simulink model "ExportExample"  (Simulink 7.6)
settings: Solver=FixedStepDiscrete  SolverMode=SingleTasking  StartTime=0.0  StopTime=100.0  RelTol=1e-3
InitFcn:
  | %% DSPBuilder Start
  | alt_dspbuilder_update_model(bdroot)
  | %% DSPBuilder End
libraries: allblocks_alteradspbuilder2 x8
settings Model: Creator=gnixon  LastModifiedBy=akarapet
settings OptimizationCC: InlineInvariantSignals=on  InitFltsAndDblsToZero=on
settings DebuggingCC: SaveWithParameterizedLinksMsg=none  SignalResolutionControl=TryResolveAllWithWarning  SolverPrmCheckMsg=none  MultiTaskDSMMsg=warning  MultiTaskCondExecSysMsg=none  StrictBusMsg=Warning
settings HardwareCC: TargetUnknown=on
settings RTWCC: IncludeERTFirstTime=on
settings GRTTargetCC: TargetFcnLib=ansi_tfl_tmw.mat

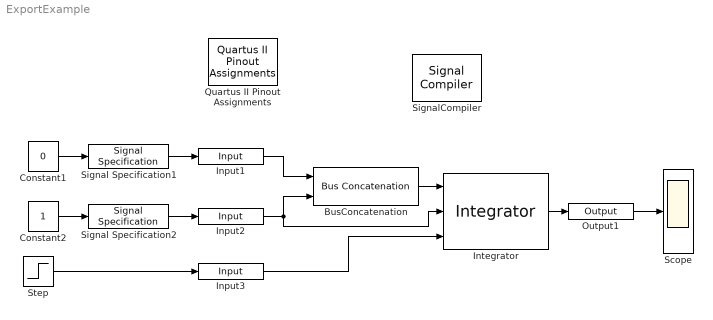
== system ExportExample ==
  BusConcatenation : allblocks_alteradspbuilder2/Bus Concatenation  isSigned=off  awidth=1  bwidth=1  pipeline_display=0
  Constant1 : Constant  Value=0
  Constant2 : Constant
  Input1 : allblocks_alteradspbuilder2/Input  iofile=/data/akarapet/qshell_linux64_test/p4/dsp_builder/dsp_builder2/Documentation/DesignExamples/Tutorials/HIL/ExportExample/tb_ExportExample/ExportExample_Input1.salt  BusType=Single Bit  bwl=1  bwr=0  SpecifyClock=off  PORTTYPE=Input  externalType=Inferred  allowFloatingPointOverride=on  logOutputs=off
  Input2 : allblocks_alteradspbuilder2/Input  iofile=/data/akarapet/qshell_linux64_test/p4/dsp_builder/dsp_builder2/Documentation/DesignExamples/Tutorials/HIL/ExportExample/tb_ExportExample/ExportExample_Input2.salt  BusType=Single Bit  bwl=1  bwr=0  SpecifyClock=off  PORTTYPE=Input  externalType=Inferred  allowFloatingPointOverride=on  logOutputs=off
  Input3 : allblocks_alteradspbuilder2/Input  iofile=/data/akarapet/qshell_linux64_test/p4/dsp_builder/dsp_builder2/Documentation/DesignExamples/Tutorials/HIL/ExportExample/tb_ExportExample/ExportExample_Input3.salt  BusType=Single Bit  bwl=1  bwr=0  SpecifyClock=off  PORTTYPE=Input  externalType=Inferred  allowFloatingPointOverride=on  logOutputs=off
  Integrator : allblocks_alteradspbuilder2/Integrator  bwl=2  depth=1  pipeline_display=1  use_ena=on  use_sclr=on  allowFloatingPointOverride=on  logOutputs=off  logFile=/data/akarapet/qshell_linux64_test/p4/dsp_builder/dsp_builder2/Documentation/DesignExamples/Tutorials/HIL/ExportExample/tb_ExportExample/ExportExample_Integrator.fixedpointlog
  Output1 : allblocks_alteradspbuilder2/Output  iofile=/data/akarapet/qshell_linux64_test/p4/dsp_builder/dsp_builder2/Documentation/DesignExamples/Tutorials/HIL/ExportExample/tb_ExportExample/ExportExample_Output1.capture  BusType=Signed Integer  bwl=2  bwr=0  externalType=Inferred  PORTTYPE=Output  allowFloatingPointOverride=on  logOutputs=off
  Quartus II Pinout Assignments : allblocks_alteradspbuilder2/Quartus II Pinout Assignments  QuartusIIAssignmentName=Input2  QuartusIIAssignmentValue=Pin_AC14
  Scope : Scope
  Signal Specification1 : SignalSpecification  SampleTime=1
  Signal Specification2 : SignalSpecification  SampleTime=1
  SignalCompiler : allblocks_alteradspbuilder2/Signal Compiler  DeviceFamily=Cyclone III  DeviceName=EP3C120F780C7  EnableSignalTap=off  SignalTapDepth=128  UseBoardBlock=off  StpUseDefaultClock=on  StpClock=Clock  ExportDir=/data/akarapet/qshell_linux64_test/p4/dsp_builder/dsp_builder2/Documentation/DesignExamples/Tutorials/HIL/ExportExample/.
  Step : Step  Time=3  Before=1  After=0  SampleTime=1
  wires:
  Constant2/1 -> Signal Specification2/1
  Constant1/1 -> Signal Specification1/1
  Integrator/1 -> Output1/1
  Signal Specification1/1 -> Input1/1
  Signal Specification2/1 -> Input2/1
  BusConcatenation/1 -> Integrator/1
  Input1/1 -> BusConcatenation/1
  Input2/1 -> BusConcatenation/2, Integrator/2
  Output1/1 -> Scope/1
  Step/1 -> Input3/1
  Input3/1 -> Integrator/3
